simulink model "IEEE34BARRAS"  (R2018a)
settings: Solver=ode4  StartTime=0.0  StopTime=48*T  FixedStep=Ts  RelTol=1e-3  EnableMultiTasking=on
InitFcn:
  | close
  | clc
  | clear
  | n=2^8;
  | f=60;
  | T=1/f;
  | Ts=1/(f*n);
  | NT=18;
  | set_param('IEEE34BARRAS/EMISOR-RECEPTOR/TCP_IP_RX1/ESCRITURA', 'Value','[0,0,0,0,0,0,0,0,0,0,0,0,0,0,0,0,0,0,0,0,0,0,0,0,0,0,0,0,0,0,0,0,0,0,0,0,0,0,0,0,0]')
  | set_param('IEEE34BARRAS/EMISOR-RECEPTOR/TCP_IP_RX1/RETARDO', 'Value','0')
  | run script_client_1_inicio1.m
undefined symbols (not defined in the file or in its folder): D1, Delta, DiscIntNeverNeededParam, Ip1
libraries: powerlib x313, simulink x15, libreria_medidores1T x3, libreria_comunicaciones_cliente1T x2
(part 4 of 5)

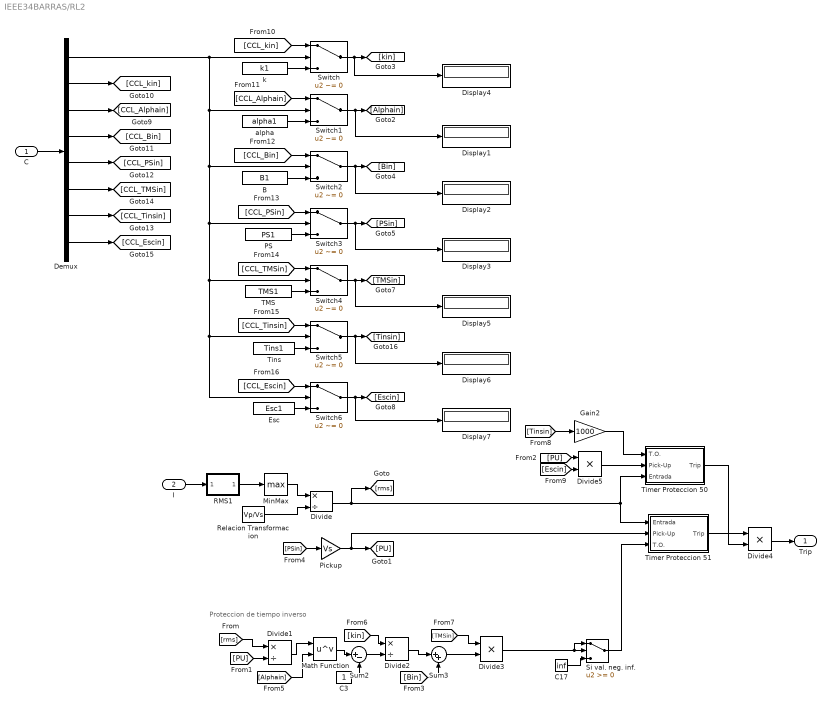
== system IEEE34BARRAS/RL2 ==
  note: Proteccion de tiempo inverso
  C : Inport
  I : Inport  Port=2
  B : Constant  Value=B1
  C17 : Constant  Value=inf
  C3 : Constant
  Demux : Demux  Outputs=8
  Display{1..7} (7 alike) : Display
  Divide : Product  Inputs=*/
  Divide1 : Product  Inputs=*/
  Divide2 : Product  Inputs=*/
  Divide3 : Product  Inputs=**
  Divide4 : Product  Inputs=**
  Divide5 : Product  Inputs=**
  Esc : Constant  Value=Esc1
  Gain2 : Gain  Gain=1000
  Math Function : Math  Operator=pow  SaturateOnIntegerOverflow=on
  MinMax : MinMax  Function=max
  PS : Constant  Value=PS1
  Pickup : Gain  Gain=Vs
  RMS1 : Subsystem
  Relacion Transformacion : Constant  Value=Vp/Vs
  Si val. neg. inf. : Switch
  Sum2 : Sum  Inputs=|+-
  Sum3 : Sum  Inputs=|++
  Switch{,1..6} (7 alike) : Switch  Criteria=u2 ~= 0
  TMS : Constant  Value=TMS1
  Timer Proteccion 50 : Subsystem
  Timer Proteccion 51 : Subsystem
  Tins : Constant  Value=Tins1
  alpha : Constant  Value=alpha1
  k : Constant  Value=k1
  Trip : Outport
  wires:
  Divide4/1 -> Trip/1
  [Escin] -> Divide5/2
  C17/1 -> Si val. neg. inf./3
  Math Function/1 -> Sum2/1
  [kin] -> Divide2/1
  Timer Proteccion 50/1(Trip) -> Divide4/2
  [PSin] -> Pickup/1
  Si val. neg. inf./1 -> Timer Proteccion 51/3(T.O.)
  [Tinsin] -> Gain2/1
  Timer Proteccion 51/1(Trip) -> Divide4/1
  [Alphain] -> Math Function/2
  [PU] -> Divide1/2
  [PU] -> Divide5/1
  Divide5/1 -> Timer Proteccion 50/2(Pick-Up)
  Divide2/1 -> Sum3/1
  Gain2/1 -> Timer Proteccion 50/1(T.O.)
  Divide3/1 -> Si val. neg. inf./1, Si val. neg. inf./2
  Sum3/1 -> Divide3/2
  [Bin] -> Sum3/2
  Relacion Transformacion/1 -> Divide/2
  Divide/1 -> Timer Proteccion 50/3(Entrada), Timer Proteccion 51/1(Entrada), [rms]
  Sum2/1 -> Divide2/2
  Divide1/1 -> Math Function/1
  [rms] -> Divide1/1
  Pickup/1 -> Timer Proteccion 51/2(Pick-Up), [PU]
  MinMax/1 -> Divide/1
  RMS1/1(Out1) -> MinMax/1
  [TMSin] -> Divide3/1
  C3/1 -> Sum2/2
  I/1 -> RMS1/1(In1)
  C/1 -> Demux/1
  Demux/1 -> Switch2/2, Switch4/2, Switch6/2, Switch5/2, Switch3/2, Switch1/2, Switch/2
  Demux/7 -> [CCL_Tinsin]
  Demux/5 -> [CCL_PSin]
  Demux/4 -> [CCL_Bin]
  Demux/2 -> [CCL_kin]
  Demux/3 -> [CCL_Alphain]
  Demux/6 -> [CCL_TMSin]
  Demux/8 -> [CCL_Escin]
  B/1 -> Switch2/3
  PS/1 -> Switch3/3
  TMS/1 -> Switch4/3
  Tins/1 -> Switch5/3
  Esc/1 -> Switch6/3
  Switch/1 -> Display4/1, [kin]
  Switch1/1 -> Display1/1, [Alphain]
  Switch3/1 -> Display3/1, [PSin]
  Switch4/1 -> Display5/1, [TMSin]
  Switch5/1 -> Display6/1, [Tinsin]
  Switch6/1 -> Display7/1, [Escin]
  alpha/1 -> Switch1/3
  [CCL_Alphain] -> Switch1/1
  [CCL_Bin] -> Switch2/1
  [CCL_PSin] -> Switch3/1
  [CCL_TMSin] -> Switch4/1
  [CCL_Tinsin] -> Switch5/1
  [CCL_Escin] -> Switch6/1
  k/1 -> Switch/3
  [CCL_kin] -> Switch/1
  Switch2/1 -> Display2/1, [Bin]

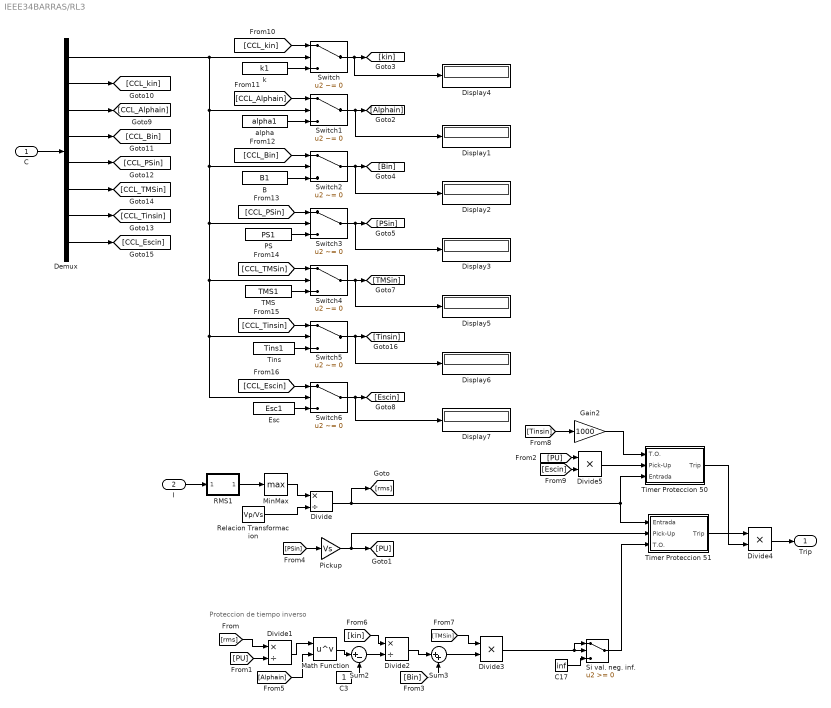
== system IEEE34BARRAS/RL3 ==
  note: Proteccion de tiempo inverso
  C : Inport
  I : Inport  Port=2
  B : Constant  Value=B1
  C17 : Constant  Value=inf
  C3 : Constant
  Demux : Demux  Outputs=8
  Display{1..7} (7 alike) : Display
  Divide : Product  Inputs=*/
  Divide1 : Product  Inputs=*/
  Divide2 : Product  Inputs=*/
  Divide3 : Product  Inputs=**
  Divide4 : Product  Inputs=**
  Divide5 : Product  Inputs=**
  Esc : Constant  Value=Esc1
  Gain2 : Gain  Gain=1000
  Math Function : Math  Operator=pow  SaturateOnIntegerOverflow=on
  MinMax : MinMax  Function=max
  PS : Constant  Value=PS1
  Pickup : Gain  Gain=Vs
  RMS1 : Subsystem
  Relacion Transformacion : Constant  Value=Vp/Vs
  Si val. neg. inf. : Switch
  Sum2 : Sum  Inputs=|+-
  Sum3 : Sum  Inputs=|++
  Switch{,1..6} (7 alike) : Switch  Criteria=u2 ~= 0
  TMS : Constant  Value=TMS1
  Timer Proteccion 50 : Subsystem
  Timer Proteccion 51 : Subsystem
  Tins : Constant  Value=Tins1
  alpha : Constant  Value=alpha1
  k : Constant  Value=k1
  Trip : Outport
  wires:
  Divide4/1 -> Trip/1
  [Escin] -> Divide5/2
  C17/1 -> Si val. neg. inf./3
  Math Function/1 -> Sum2/1
  [kin] -> Divide2/1
  Timer Proteccion 50/1(Trip) -> Divide4/2
  [PSin] -> Pickup/1
  Si val. neg. inf./1 -> Timer Proteccion 51/3(T.O.)
  [Tinsin] -> Gain2/1
  Timer Proteccion 51/1(Trip) -> Divide4/1
  [Alphain] -> Math Function/2
  [PU] -> Divide1/2
  [PU] -> Divide5/1
  Divide5/1 -> Timer Proteccion 50/2(Pick-Up)
  Divide2/1 -> Sum3/1
  Gain2/1 -> Timer Proteccion 50/1(T.O.)
  Divide3/1 -> Si val. neg. inf./1, Si val. neg. inf./2
  Sum3/1 -> Divide3/2
  [Bin] -> Sum3/2
  Relacion Transformacion/1 -> Divide/2
  Divide/1 -> Timer Proteccion 50/3(Entrada), Timer Proteccion 51/1(Entrada), [rms]
  Sum2/1 -> Divide2/2
  Divide1/1 -> Math Function/1
  [rms] -> Divide1/1
  Pickup/1 -> Timer Proteccion 51/2(Pick-Up), [PU]
  MinMax/1 -> Divide/1
  RMS1/1(Out1) -> MinMax/1
  [TMSin] -> Divide3/1
  C3/1 -> Sum2/2
  I/1 -> RMS1/1(In1)
  C/1 -> Demux/1
  Demux/1 -> Switch2/2, Switch4/2, Switch6/2, Switch5/2, Switch3/2, Switch1/2, Switch/2
  Demux/7 -> [CCL_Tinsin]
  Demux/5 -> [CCL_PSin]
  Demux/4 -> [CCL_Bin]
  Demux/2 -> [CCL_kin]
  Demux/3 -> [CCL_Alphain]
  Demux/6 -> [CCL_TMSin]
  Demux/8 -> [CCL_Escin]
  B/1 -> Switch2/3
  PS/1 -> Switch3/3
  TMS/1 -> Switch4/3
  Tins/1 -> Switch5/3
  Esc/1 -> Switch6/3
  Switch/1 -> Display4/1, [kin]
  Switch1/1 -> Display1/1, [Alphain]
  Switch3/1 -> Display3/1, [PSin]
  Switch4/1 -> Display5/1, [TMSin]
  Switch5/1 -> Display6/1, [Tinsin]
  Switch6/1 -> Display7/1, [Escin]
  alpha/1 -> Switch1/3
  [CCL_Alphain] -> Switch1/1
  [CCL_Bin] -> Switch2/1
  [CCL_PSin] -> Switch3/1
  [CCL_TMSin] -> Switch4/1
  [CCL_Tinsin] -> Switch5/1
  [CCL_Escin] -> Switch6/1
  k/1 -> Switch/3
  [CCL_kin] -> Switch/1
  Switch2/1 -> Display2/1, [Bin]

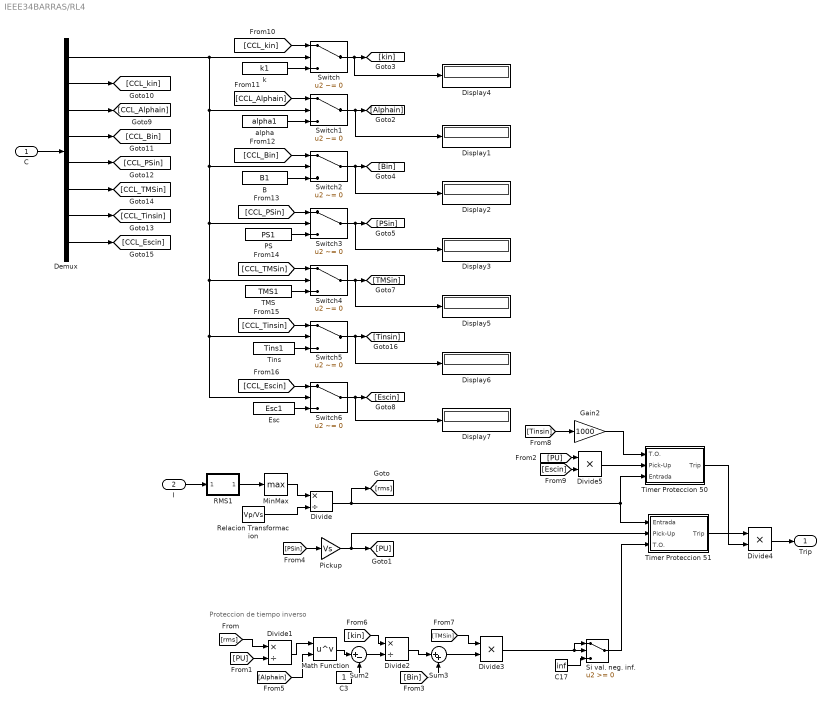
== system IEEE34BARRAS/RL4 ==
  note: Proteccion de tiempo inverso
  C : Inport
  I : Inport  Port=2
  B : Constant  Value=B1
  C17 : Constant  Value=inf
  C3 : Constant
  Demux : Demux  Outputs=8
  Display{1..7} (7 alike) : Display
  Divide : Product  Inputs=*/
  Divide1 : Product  Inputs=*/
  Divide2 : Product  Inputs=*/
  Divide3 : Product  Inputs=**
  Divide4 : Product  Inputs=**
  Divide5 : Product  Inputs=**
  Esc : Constant  Value=Esc1
  Gain2 : Gain  Gain=1000
  Math Function : Math  Operator=pow  SaturateOnIntegerOverflow=on
  MinMax : MinMax  Function=max
  PS : Constant  Value=PS1
  Pickup : Gain  Gain=Vs
  RMS1 : Subsystem
  Relacion Transformacion : Constant  Value=Vp/Vs
  Si val. neg. inf. : Switch
  Sum2 : Sum  Inputs=|+-
  Sum3 : Sum  Inputs=|++
  Switch{,1..6} (7 alike) : Switch  Criteria=u2 ~= 0
  TMS : Constant  Value=TMS1
  Timer Proteccion 50 : Subsystem
  Timer Proteccion 51 : Subsystem
  Tins : Constant  Value=Tins1
  alpha : Constant  Value=alpha1
  k : Constant  Value=k1
  Trip : Outport
  wires:
  Divide4/1 -> Trip/1
  [Escin] -> Divide5/2
  C17/1 -> Si val. neg. inf./3
  Math Function/1 -> Sum2/1
  [kin] -> Divide2/1
  Timer Proteccion 50/1(Trip) -> Divide4/2
  [PSin] -> Pickup/1
  Si val. neg. inf./1 -> Timer Proteccion 51/3(T.O.)
  [Tinsin] -> Gain2/1
  Timer Proteccion 51/1(Trip) -> Divide4/1
  [Alphain] -> Math Function/2
  [PU] -> Divide1/2
  [PU] -> Divide5/1
  Divide5/1 -> Timer Proteccion 50/2(Pick-Up)
  Divide2/1 -> Sum3/1
  Gain2/1 -> Timer Proteccion 50/1(T.O.)
  Divide3/1 -> Si val. neg. inf./1, Si val. neg. inf./2
  Sum3/1 -> Divide3/2
  [Bin] -> Sum3/2
  Relacion Transformacion/1 -> Divide/2
  Divide/1 -> Timer Proteccion 50/3(Entrada), Timer Proteccion 51/1(Entrada), [rms]
  Sum2/1 -> Divide2/2
  Divide1/1 -> Math Function/1
  [rms] -> Divide1/1
  Pickup/1 -> Timer Proteccion 51/2(Pick-Up), [PU]
  MinMax/1 -> Divide/1
  RMS1/1(Out1) -> MinMax/1
  [TMSin] -> Divide3/1
  C3/1 -> Sum2/2
  I/1 -> RMS1/1(In1)
  C/1 -> Demux/1
  Demux/1 -> Switch2/2, Switch4/2, Switch6/2, Switch5/2, Switch3/2, Switch1/2, Switch/2
  Demux/7 -> [CCL_Tinsin]
  Demux/5 -> [CCL_PSin]
  Demux/4 -> [CCL_Bin]
  Demux/2 -> [CCL_kin]
  Demux/3 -> [CCL_Alphain]
  Demux/6 -> [CCL_TMSin]
  Demux/8 -> [CCL_Escin]
  B/1 -> Switch2/3
  PS/1 -> Switch3/3
  TMS/1 -> Switch4/3
  Tins/1 -> Switch5/3
  Esc/1 -> Switch6/3
  Switch/1 -> Display4/1, [kin]
  Switch1/1 -> Display1/1, [Alphain]
  Switch3/1 -> Display3/1, [PSin]
  Switch4/1 -> Display5/1, [TMSin]
  Switch5/1 -> Display6/1, [Tinsin]
  Switch6/1 -> Display7/1, [Escin]
  alpha/1 -> Switch1/3
  [CCL_Alphain] -> Switch1/1
  [CCL_Bin] -> Switch2/1
  [CCL_PSin] -> Switch3/1
  [CCL_TMSin] -> Switch4/1
  [CCL_Tinsin] -> Switch5/1
  [CCL_Escin] -> Switch6/1
  k/1 -> Switch/3
  [CCL_kin] -> Switch/1
  Switch2/1 -> Display2/1, [Bin]

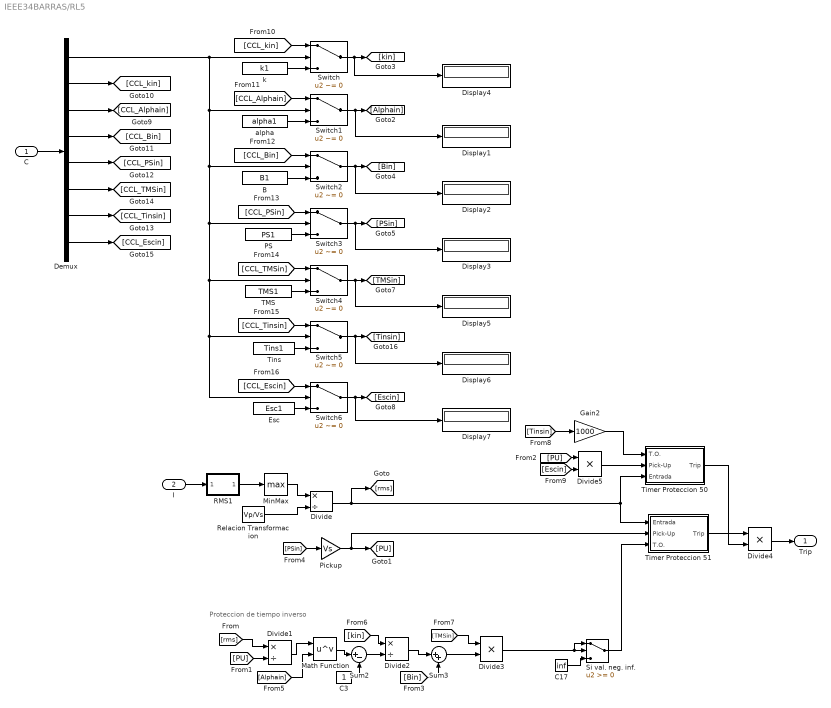
== system IEEE34BARRAS/RL5 ==
  note: Proteccion de tiempo inverso
  C : Inport
  I : Inport  Port=2
  B : Constant  Value=B1
  C17 : Constant  Value=inf
  C3 : Constant
  Demux : Demux  Outputs=8
  Display{1..7} (7 alike) : Display
  Divide : Product  Inputs=*/
  Divide1 : Product  Inputs=*/
  Divide2 : Product  Inputs=*/
  Divide3 : Product  Inputs=**
  Divide4 : Product  Inputs=**
  Divide5 : Product  Inputs=**
  Esc : Constant  Value=Esc1
  Gain2 : Gain  Gain=1000
  Math Function : Math  Operator=pow  SaturateOnIntegerOverflow=on
  MinMax : MinMax  Function=max
  PS : Constant  Value=PS1
  Pickup : Gain  Gain=Vs
  RMS1 : Subsystem
  Relacion Transformacion : Constant  Value=Vp/Vs
  Si val. neg. inf. : Switch
  Sum2 : Sum  Inputs=|+-
  Sum3 : Sum  Inputs=|++
  Switch{,1..6} (7 alike) : Switch  Criteria=u2 ~= 0
  TMS : Constant  Value=TMS1
  Timer Proteccion 50 : Subsystem
  Timer Proteccion 51 : Subsystem
  Tins : Constant  Value=Tins1
  alpha : Constant  Value=alpha1
  k : Constant  Value=k1
  Trip : Outport
  wires:
  Divide4/1 -> Trip/1
  [Escin] -> Divide5/2
  C17/1 -> Si val. neg. inf./3
  Math Function/1 -> Sum2/1
  [kin] -> Divide2/1
  Timer Proteccion 50/1(Trip) -> Divide4/2
  [PSin] -> Pickup/1
  Si val. neg. inf./1 -> Timer Proteccion 51/3(T.O.)
  [Tinsin] -> Gain2/1
  Timer Proteccion 51/1(Trip) -> Divide4/1
  [Alphain] -> Math Function/2
  [PU] -> Divide1/2
  [PU] -> Divide5/1
  Divide5/1 -> Timer Proteccion 50/2(Pick-Up)
  Divide2/1 -> Sum3/1
  Gain2/1 -> Timer Proteccion 50/1(T.O.)
  Divide3/1 -> Si val. neg. inf./1, Si val. neg. inf./2
  Sum3/1 -> Divide3/2
  [Bin] -> Sum3/2
  Relacion Transformacion/1 -> Divide/2
  Divide/1 -> Timer Proteccion 50/3(Entrada), Timer Proteccion 51/1(Entrada), [rms]
  Sum2/1 -> Divide2/2
  Divide1/1 -> Math Function/1
  [rms] -> Divide1/1
  Pickup/1 -> Timer Proteccion 51/2(Pick-Up), [PU]
  MinMax/1 -> Divide/1
  RMS1/1(Out1) -> MinMax/1
  [TMSin] -> Divide3/1
  C3/1 -> Sum2/2
  I/1 -> RMS1/1(In1)
  C/1 -> Demux/1
  Demux/1 -> Switch2/2, Switch4/2, Switch6/2, Switch5/2, Switch3/2, Switch1/2, Switch/2
  Demux/7 -> [CCL_Tinsin]
  Demux/5 -> [CCL_PSin]
  Demux/4 -> [CCL_Bin]
  Demux/2 -> [CCL_kin]
  Demux/3 -> [CCL_Alphain]
  Demux/6 -> [CCL_TMSin]
  Demux/8 -> [CCL_Escin]
  B/1 -> Switch2/3
  PS/1 -> Switch3/3
  TMS/1 -> Switch4/3
  Tins/1 -> Switch5/3
  Esc/1 -> Switch6/3
  Switch/1 -> Display4/1, [kin]
  Switch1/1 -> Display1/1, [Alphain]
  Switch3/1 -> Display3/1, [PSin]
  Switch4/1 -> Display5/1, [TMSin]
  Switch5/1 -> Display6/1, [Tinsin]
  Switch6/1 -> Display7/1, [Escin]
  alpha/1 -> Switch1/3
  [CCL_Alphain] -> Switch1/1
  [CCL_Bin] -> Switch2/1
  [CCL_PSin] -> Switch3/1
  [CCL_TMSin] -> Switch4/1
  [CCL_Tinsin] -> Switch5/1
  [CCL_Escin] -> Switch6/1
  k/1 -> Switch/3
  [CCL_kin] -> Switch/1
  Switch2/1 -> Display2/1, [Bin]

== system IEEE34BARRAS/Subsystem4 ==
  3p : powerlib/Elements/Three-Phase Fault  InitialStates=0  FaultA=on  FaultB=on  FaultC=on  GroundFault=on  SwitchTimes=[30*T]  External=off  SwitchStatus=NaN  FaultResistance=0.001  GroundResistance=1  SnubberResistance=1e6  SnubberCapacitance=inf  Measurements=None
  Conn1 : PMIOPort  Side=Left
  Conn2 : PMIOPort  Port=2  Side=Left
  Conn3 : PMIOPort  Port=3  Side=Left
  connections:
  3p/LConn3 -- Conn3/RConn1
  3p/LConn1 -- Conn1/RConn1
  3p/LConn2 -- Conn2/RConn1

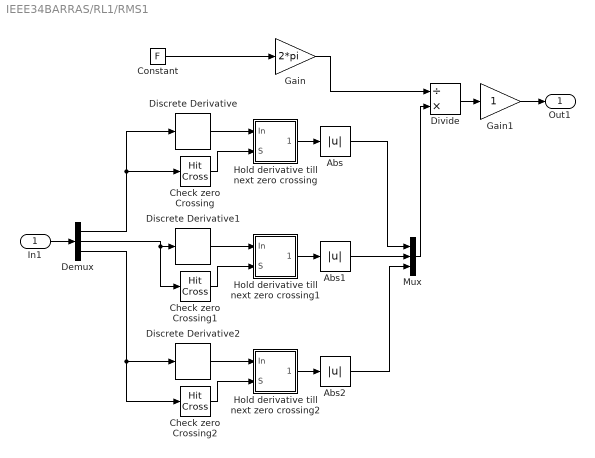
== system IEEE34BARRAS/RL1/RMS1 ==
  In1 : Inport
  Abs : Abs
  Abs1 : Abs
  Abs2 : Abs
  Check zero Crossing : HitCross
  Check zero Crossing1 : HitCross
  Check zero Crossing2 : HitCross
  Constant : Constant  Value=F
  Demux : Demux  Outputs=3
  Discrete Derivative : simulink/Discrete/Discrete Derivative  gainval=1.0  ICPrevScaledInput=0.0  OutMin=[]  OutMax=[]  OutDataType=fixdt(1, 16)  OutScaling=2^-10  DoSatur=off
  Discrete Derivative1 : simulink/Discrete/Discrete Derivative  gainval=1.0  ICPrevScaledInput=0.0  OutMin=[]  OutMax=[]  OutDataType=fixdt(1, 16)  OutScaling=2^-10  DoSatur=off
  Discrete Derivative2 : simulink/Discrete/Discrete Derivative  gainval=1.0  ICPrevScaledInput=0.0  OutMin=[]  OutMax=[]  OutDataType=fixdt(1, 16)  OutScaling=2^-10  DoSatur=off
  Divide : Product  Inputs=/*
  Gain : Gain  Gain=2*pi
  Gain1 : Gain
  Hold derivative till next zero crossing : Subsystem  AncestorBlock=|  DialogController=POWERSYS.PowerSysDialog  mask(Discrete Sample & Hold){ic=0, Ts=-1}
      | powerlib_extras/Discrete 
      | Control Blocks/Discrete
      | Sample & Hold
      mask prompts: ic "Initial condition:"; Ts "Sample time:"
      mask help: The output follows input 1 (In) as long as input 2 (S) is TRUE (1) . The output is held when input 2 becomes FALSE (0). The output initial value is specified by the parameter "Initial condition".
      mask init:
      | power_initmask();
      mask Help: This block is part of a subset of blocks in the Extras library that does not have documentation associated with it, other than the block mask description.
      mask Display: disp('S/H')
  Hold derivative till next zero crossing1 : Subsystem  AncestorBlock=|  DialogController=POWERSYS.PowerSysDialog  mask(Discrete Sample & Hold){ic=0, Ts=-1}
      | powerlib_extras/Discrete 
      | Control Blocks/Discrete
      | Sample & Hold
      mask prompts: ic "Initial condition:"; Ts "Sample time:"
      mask help: The output follows input 1 (In) as long as input 2 (S) is TRUE (1) . The output is held when input 2 becomes FALSE (0). The output initial value is specified by the parameter "Initial condition".
      mask init:
      | power_initmask();
      mask Help: This block is part of a subset of blocks in the Extras library that does not have documentation associated with it, other than the block mask description.
      mask Display: disp('S/H')
  Hold derivative till next zero crossing2 : Subsystem  AncestorBlock=|  DialogController=POWERSYS.PowerSysDialog  mask(Discrete Sample & Hold){ic=0, Ts=-1}
      | powerlib_extras/Discrete 
      | Control Blocks/Discrete
      | Sample & Hold
      mask prompts: ic "Initial condition:"; Ts "Sample time:"
      mask help: The output follows input 1 (In) as long as input 2 (S) is TRUE (1) . The output is held when input 2 becomes FALSE (0). The output initial value is specified by the parameter "Initial condition".
      mask init:
      | power_initmask();
      mask Help: This block is part of a subset of blocks in the Extras library that does not have documentation associated with it, other than the block mask description.
      mask Display: disp('S/H')
  Mux : Mux  Inputs=3
  Out1 : Outport
  wires:
  Discrete Derivative/1 -> Hold derivative till next zero crossing/1(In)
  Check zero Crossing/1 -> Hold derivative till next zero crossing/2(S)
  Hold derivative till next zero crossing/1("   ") -> Abs/1
  Constant/1 -> Gain/1
  Gain/1 -> Divide/1
  Abs/1 -> Mux/1
  Demux/1 -> Check zero Crossing/1, Discrete Derivative/1
  Divide/1 -> Gain1/1
  Gain1/1 -> Out1/1
  Hold derivative till next zero crossing1/1("   ") -> Abs1/1
  Check zero Crossing1/1 -> Hold derivative till next zero crossing1/2(S)
  Discrete Derivative1/1 -> Hold derivative till next zero crossing1/1(In)
  Discrete Derivative2/1 -> Hold derivative till next zero crossing2/1(In)
  Check zero Crossing2/1 -> Hold derivative till next zero crossing2/2(S)
  Hold derivative till next zero crossing2/1("   ") -> Abs2/1
  Demux/2 -> Check zero Crossing1/1, Discrete Derivative1/1
  Demux/3 -> Check zero Crossing2/1, Discrete Derivative2/1
  Abs1/1 -> Mux/2
  Mux/1 -> Divide/2
  Abs2/1 -> Mux/3
  In1/1 -> Demux/1

== system IEEE34BARRAS/RL1/Timer Proteccion 50 ==
  T.O. : Inport
  Pick-Up : Inport  Port=2
  Entrada : Inport  Port=3
  Arranq3 : Switch  Criteria=u2 ~= 0  Threshold=Ip1
  Arranq6 : Switch  Criteria=u2 ~= 0  Threshold=Ip1  ZeroCross=off
  C14 : Constant  Value=0
  C15 : Constant  Value=1000
  C16 : Constant
  Condicion arranque1 : RelationalOperator  Operator=>  OutDataTypeStr=boolean  RndMeth=Nearest
  Discrete-Time Integrator : DiscreteIntegrator  ExternalReset=falling  SampleTime=-1  ICPrevOutput=DiscIntNeverNeededParam  ICPrevScaledInput=DiscIntNeverNeededParam
  Logical Operator4 : Logic  Operator=NOT  AllPortsSameDT=off  OutDataTypeStr=boolean
  Tiempo Disparo1 : RelationalOperator  OutDataTypeStr=boolean  RndMeth=Nearest
  Trip : Outport
  wires:
  C16/1 -> Arranq6/1
  Arranq6/1 -> Logical Operator4/1, Arranq6/3
  Tiempo Disparo1/1 -> Arranq6/2
  C15/1 -> Arranq3/1
  C14/1 -> Arranq3/3
  Arranq3/1 -> Discrete-Time Integrator/1
  Condicion arranque1/1 -> Arranq3/2, Discrete-Time Integrator/2
  Pick-Up/1 -> Condicion arranque1/2
  Discrete-Time Integrator/1 -> Tiempo Disparo1/1
  Logical Operator4/1 -> Trip/1
  Entrada/1 -> Condicion arranque1/1
  T.O./1 -> Tiempo Disparo1/2

== system IEEE34BARRAS/RL1/Timer Proteccion 51 ==
  Entrada : Inport
  Pick-Up : Inport  Port=2
  T.O. : Inport  Port=3
  Arranq3 : Switch  Criteria=u2 ~= 0  Threshold=Ip1
  Arranq6 : Switch  Criteria=u2 ~= 0  Threshold=Ip1  ZeroCross=off
  C14 : Constant  Value=0
  C15 : Constant
  C16 : Constant
  Condicion arranque1 : RelationalOperator  Operator=>  OutDataTypeStr=boolean  RndMeth=Nearest
  Discrete-Time Integrator : DiscreteIntegrator  gainval=1  ExternalReset=falling  SampleTime=-1  ICPrevOutput=DiscIntNeverNeededParam  ICPrevScaledInput=DiscIntNeverNeededParam
  Logical Operator4 : Logic  Operator=NOT  AllPortsSameDT=off  OutDataTypeStr=boolean
  Tiempo Disparo1 : RelationalOperator  OutDataTypeStr=boolean  RndMeth=Nearest
  Trip : Outport
  wires:
  C16/1 -> Arranq6/1
  Arranq6/1 -> Logical Operator4/1, Arranq6/3
  Tiempo Disparo1/1 -> Arranq6/2
  T.O./1 -> Tiempo Disparo1/2
  C15/1 -> Arranq3/1
  C14/1 -> Arranq3/3
  Arranq3/1 -> Discrete-Time Integrator/1
  Condicion arranque1/1 -> Arranq3/2, Discrete-Time Integrator/2
  Pick-Up/1 -> Condicion arranque1/2
  Entrada/1 -> Condicion arranque1/1
  Discrete-Time Integrator/1 -> Tiempo Disparo1/1
  Logical Operator4/1 -> Trip/1

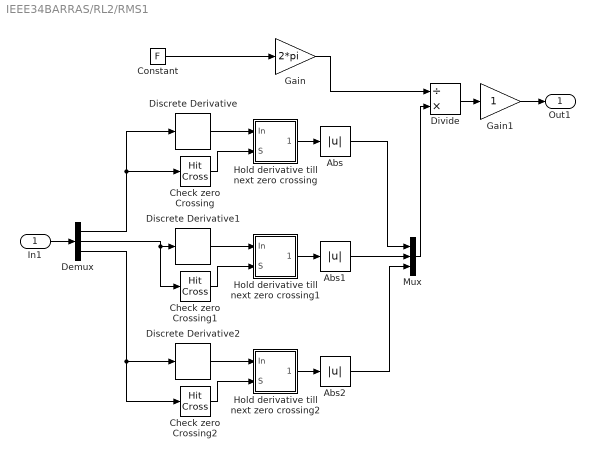
== system IEEE34BARRAS/RL2/RMS1 ==
  In1 : Inport
  Abs : Abs
  Abs1 : Abs
  Abs2 : Abs
  Check zero Crossing : HitCross
  Check zero Crossing1 : HitCross
  Check zero Crossing2 : HitCross
  Constant : Constant  Value=F
  Demux : Demux  Outputs=3
  Discrete Derivative : simulink/Discrete/Discrete Derivative  gainval=1.0  ICPrevScaledInput=0.0  OutMin=[]  OutMax=[]  OutDataType=fixdt(1, 16)  OutScaling=2^-10  DoSatur=off
  Discrete Derivative1 : simulink/Discrete/Discrete Derivative  gainval=1.0  ICPrevScaledInput=0.0  OutMin=[]  OutMax=[]  OutDataType=fixdt(1, 16)  OutScaling=2^-10  DoSatur=off
  Discrete Derivative2 : simulink/Discrete/Discrete Derivative  gainval=1.0  ICPrevScaledInput=0.0  OutMin=[]  OutMax=[]  OutDataType=fixdt(1, 16)  OutScaling=2^-10  DoSatur=off
  Divide : Product  Inputs=/*
  Gain : Gain  Gain=2*pi
  Gain1 : Gain
  Hold derivative till next zero crossing : Subsystem  AncestorBlock=|  DialogController=POWERSYS.PowerSysDialog  mask(Discrete Sample & Hold){ic=0, Ts=-1}
      | powerlib_extras/Discrete 
      | Control Blocks/Discrete
      | Sample & Hold
      mask prompts: ic "Initial condition:"; Ts "Sample time:"
      mask help: The output follows input 1 (In) as long as input 2 (S) is TRUE (1) . The output is held when input 2 becomes FALSE (0). The output initial value is specified by the parameter "Initial condition".
      mask init:
      | power_initmask();
      mask Help: This block is part of a subset of blocks in the Extras library that does not have documentation associated with it, other than the block mask description.
      mask Display: disp('S/H')
  Hold derivative till next zero crossing1 : Subsystem  AncestorBlock=|  DialogController=POWERSYS.PowerSysDialog  mask(Discrete Sample & Hold){ic=0, Ts=-1}
      | powerlib_extras/Discrete 
      | Control Blocks/Discrete
      | Sample & Hold
      mask prompts: ic "Initial condition:"; Ts "Sample time:"
      mask help: The output follows input 1 (In) as long as input 2 (S) is TRUE (1) . The output is held when input 2 becomes FALSE (0). The output initial value is specified by the parameter "Initial condition".
      mask init:
      | power_initmask();
      mask Help: This block is part of a subset of blocks in the Extras library that does not have documentation associated with it, other than the block mask description.
      mask Display: disp('S/H')
  Hold derivative till next zero crossing2 : Subsystem  AncestorBlock=|  DialogController=POWERSYS.PowerSysDialog  mask(Discrete Sample & Hold){ic=0, Ts=-1}
      | powerlib_extras/Discrete 
      | Control Blocks/Discrete
      | Sample & Hold
      mask prompts: ic "Initial condition:"; Ts "Sample time:"
      mask help: The output follows input 1 (In) as long as input 2 (S) is TRUE (1) . The output is held when input 2 becomes FALSE (0). The output initial value is specified by the parameter "Initial condition".
      mask init:
      | power_initmask();
      mask Help: This block is part of a subset of blocks in the Extras library that does not have documentation associated with it, other than the block mask description.
      mask Display: disp('S/H')
  Mux : Mux  Inputs=3
  Out1 : Outport
  wires:
  Discrete Derivative/1 -> Hold derivative till next zero crossing/1(In)
  Check zero Crossing/1 -> Hold derivative till next zero crossing/2(S)
  Hold derivative till next zero crossing/1("   ") -> Abs/1
  Constant/1 -> Gain/1
  Gain/1 -> Divide/1
  Abs/1 -> Mux/1
  Demux/1 -> Check zero Crossing/1, Discrete Derivative/1
  Divide/1 -> Gain1/1
  Gain1/1 -> Out1/1
  Hold derivative till next zero crossing1/1("   ") -> Abs1/1
  Check zero Crossing1/1 -> Hold derivative till next zero crossing1/2(S)
  Discrete Derivative1/1 -> Hold derivative till next zero crossing1/1(In)
  Discrete Derivative2/1 -> Hold derivative till next zero crossing2/1(In)
  Check zero Crossing2/1 -> Hold derivative till next zero crossing2/2(S)
  Hold derivative till next zero crossing2/1("   ") -> Abs2/1
  Demux/2 -> Check zero Crossing1/1, Discrete Derivative1/1
  Demux/3 -> Check zero Crossing2/1, Discrete Derivative2/1
  Abs1/1 -> Mux/2
  Mux/1 -> Divide/2
  Abs2/1 -> Mux/3
  In1/1 -> Demux/1

== system IEEE34BARRAS/RL2/Timer Proteccion 50 ==
  T.O. : Inport
  Pick-Up : Inport  Port=2
  Entrada : Inport  Port=3
  Arranq3 : Switch  Criteria=u2 ~= 0  Threshold=Ip1
  Arranq6 : Switch  Criteria=u2 ~= 0  Threshold=Ip1  ZeroCross=off
  C14 : Constant  Value=0
  C15 : Constant  Value=1000
  C16 : Constant
  Condicion arranque1 : RelationalOperator  Operator=>  OutDataTypeStr=boolean  RndMeth=Nearest
  Discrete-Time Integrator : DiscreteIntegrator  ExternalReset=falling  SampleTime=-1  ICPrevOutput=DiscIntNeverNeededParam  ICPrevScaledInput=DiscIntNeverNeededParam
  Logical Operator4 : Logic  Operator=NOT  AllPortsSameDT=off  OutDataTypeStr=boolean
  Tiempo Disparo1 : RelationalOperator  OutDataTypeStr=boolean  RndMeth=Nearest
  Trip : Outport
  wires:
  C16/1 -> Arranq6/1
  Arranq6/1 -> Logical Operator4/1, Arranq6/3
  Tiempo Disparo1/1 -> Arranq6/2
  C15/1 -> Arranq3/1
  C14/1 -> Arranq3/3
  Arranq3/1 -> Discrete-Time Integrator/1
  Condicion arranque1/1 -> Arranq3/2, Discrete-Time Integrator/2
  Pick-Up/1 -> Condicion arranque1/2
  Discrete-Time Integrator/1 -> Tiempo Disparo1/1
  Logical Operator4/1 -> Trip/1
  Entrada/1 -> Condicion arranque1/1
  T.O./1 -> Tiempo Disparo1/2

== system IEEE34BARRAS/RL2/Timer Proteccion 51 ==
  Entrada : Inport
  Pick-Up : Inport  Port=2
  T.O. : Inport  Port=3
  Arranq3 : Switch  Criteria=u2 ~= 0  Threshold=Ip1
  Arranq6 : Switch  Criteria=u2 ~= 0  Threshold=Ip1  ZeroCross=off
  C14 : Constant  Value=0
  C15 : Constant
  C16 : Constant
  Condicion arranque1 : RelationalOperator  Operator=>  OutDataTypeStr=boolean  RndMeth=Nearest
  Discrete-Time Integrator : DiscreteIntegrator  gainval=1  ExternalReset=falling  SampleTime=-1  ICPrevOutput=DiscIntNeverNeededParam  ICPrevScaledInput=DiscIntNeverNeededParam
  Logical Operator4 : Logic  Operator=NOT  AllPortsSameDT=off  OutDataTypeStr=boolean
  Tiempo Disparo1 : RelationalOperator  OutDataTypeStr=boolean  RndMeth=Nearest
  Trip : Outport
  wires:
  C16/1 -> Arranq6/1
  Arranq6/1 -> Logical Operator4/1, Arranq6/3
  Tiempo Disparo1/1 -> Arranq6/2
  T.O./1 -> Tiempo Disparo1/2
  C15/1 -> Arranq3/1
  C14/1 -> Arranq3/3
  Arranq3/1 -> Discrete-Time Integrator/1
  Condicion arranque1/1 -> Arranq3/2, Discrete-Time Integrator/2
  Pick-Up/1 -> Condicion arranque1/2
  Entrada/1 -> Condicion arranque1/1
  Discrete-Time Integrator/1 -> Tiempo Disparo1/1
  Logical Operator4/1 -> Trip/1

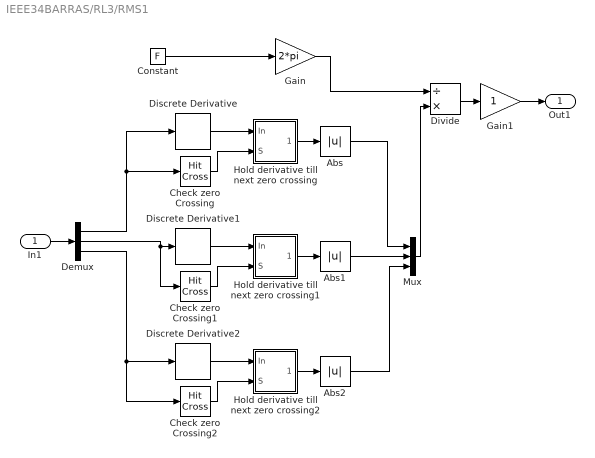
== system IEEE34BARRAS/RL3/RMS1 ==
  In1 : Inport
  Abs : Abs
  Abs1 : Abs
  Abs2 : Abs
  Check zero Crossing : HitCross
  Check zero Crossing1 : HitCross
  Check zero Crossing2 : HitCross
  Constant : Constant  Value=F
  Demux : Demux  Outputs=3
  Discrete Derivative : simulink/Discrete/Discrete Derivative  gainval=1.0  ICPrevScaledInput=0.0  OutMin=[]  OutMax=[]  OutDataType=fixdt(1, 16)  OutScaling=2^-10  DoSatur=off
  Discrete Derivative1 : simulink/Discrete/Discrete Derivative  gainval=1.0  ICPrevScaledInput=0.0  OutMin=[]  OutMax=[]  OutDataType=fixdt(1, 16)  OutScaling=2^-10  DoSatur=off
  Discrete Derivative2 : simulink/Discrete/Discrete Derivative  gainval=1.0  ICPrevScaledInput=0.0  OutMin=[]  OutMax=[]  OutDataType=fixdt(1, 16)  OutScaling=2^-10  DoSatur=off
  Divide : Product  Inputs=/*
  Gain : Gain  Gain=2*pi
  Gain1 : Gain
  Hold derivative till next zero crossing : Subsystem  AncestorBlock=|  DialogController=POWERSYS.PowerSysDialog  mask(Discrete Sample & Hold){ic=0, Ts=-1}
      | powerlib_extras/Discrete 
      | Control Blocks/Discrete
      | Sample & Hold
      mask prompts: ic "Initial condition:"; Ts "Sample time:"
      mask help: The output follows input 1 (In) as long as input 2 (S) is TRUE (1) . The output is held when input 2 becomes FALSE (0). The output initial value is specified by the parameter "Initial condition".
      mask init:
      | power_initmask();
      mask Help: This block is part of a subset of blocks in the Extras library that does not have documentation associated with it, other than the block mask description.
      mask Display: disp('S/H')
  Hold derivative till next zero crossing1 : Subsystem  AncestorBlock=|  DialogController=POWERSYS.PowerSysDialog  mask(Discrete Sample & Hold){ic=0, Ts=-1}
      | powerlib_extras/Discrete 
      | Control Blocks/Discrete
      | Sample & Hold
      mask prompts: ic "Initial condition:"; Ts "Sample time:"
      mask help: The output follows input 1 (In) as long as input 2 (S) is TRUE (1) . The output is held when input 2 becomes FALSE (0). The output initial value is specified by the parameter "Initial condition".
      mask init:
      | power_initmask();
      mask Help: This block is part of a subset of blocks in the Extras library that does not have documentation associated with it, other than the block mask description.
      mask Display: disp('S/H')
  Hold derivative till next zero crossing2 : Subsystem  AncestorBlock=|  DialogController=POWERSYS.PowerSysDialog  mask(Discrete Sample & Hold){ic=0, Ts=-1}
      | powerlib_extras/Discrete 
      | Control Blocks/Discrete
      | Sample & Hold
      mask prompts: ic "Initial condition:"; Ts "Sample time:"
      mask help: The output follows input 1 (In) as long as input 2 (S) is TRUE (1) . The output is held when input 2 becomes FALSE (0). The output initial value is specified by the parameter "Initial condition".
      mask init:
      | power_initmask();
      mask Help: This block is part of a subset of blocks in the Extras library that does not have documentation associated with it, other than the block mask description.
      mask Display: disp('S/H')
  Mux : Mux  Inputs=3
  Out1 : Outport
  wires:
  Discrete Derivative/1 -> Hold derivative till next zero crossing/1(In)
  Check zero Crossing/1 -> Hold derivative till next zero crossing/2(S)
  Hold derivative till next zero crossing/1("   ") -> Abs/1
  Constant/1 -> Gain/1
  Gain/1 -> Divide/1
  Abs/1 -> Mux/1
  Demux/1 -> Check zero Crossing/1, Discrete Derivative/1
  Divide/1 -> Gain1/1
  Gain1/1 -> Out1/1
  Hold derivative till next zero crossing1/1("   ") -> Abs1/1
  Check zero Crossing1/1 -> Hold derivative till next zero crossing1/2(S)
  Discrete Derivative1/1 -> Hold derivative till next zero crossing1/1(In)
  Discrete Derivative2/1 -> Hold derivative till next zero crossing2/1(In)
  Check zero Crossing2/1 -> Hold derivative till next zero crossing2/2(S)
  Hold derivative till next zero crossing2/1("   ") -> Abs2/1
  Demux/2 -> Check zero Crossing1/1, Discrete Derivative1/1
  Demux/3 -> Check zero Crossing2/1, Discrete Derivative2/1
  Abs1/1 -> Mux/2
  Mux/1 -> Divide/2
  Abs2/1 -> Mux/3
  In1/1 -> Demux/1

== system IEEE34BARRAS/RL3/Timer Proteccion 50 ==
  T.O. : Inport
  Pick-Up : Inport  Port=2
  Entrada : Inport  Port=3
  Arranq3 : Switch  Criteria=u2 ~= 0  Threshold=Ip1
  Arranq6 : Switch  Criteria=u2 ~= 0  Threshold=Ip1  ZeroCross=off
  C14 : Constant  Value=0
  C15 : Constant  Value=1000
  C16 : Constant
  Condicion arranque1 : RelationalOperator  Operator=>  OutDataTypeStr=boolean  RndMeth=Nearest
  Discrete-Time Integrator : DiscreteIntegrator  ExternalReset=falling  SampleTime=-1  ICPrevOutput=DiscIntNeverNeededParam  ICPrevScaledInput=DiscIntNeverNeededParam
  Logical Operator4 : Logic  Operator=NOT  AllPortsSameDT=off  OutDataTypeStr=boolean
  Tiempo Disparo1 : RelationalOperator  OutDataTypeStr=boolean  RndMeth=Nearest
  Trip : Outport
  wires:
  C16/1 -> Arranq6/1
  Arranq6/1 -> Logical Operator4/1, Arranq6/3
  Tiempo Disparo1/1 -> Arranq6/2
  C15/1 -> Arranq3/1
  C14/1 -> Arranq3/3
  Arranq3/1 -> Discrete-Time Integrator/1
  Condicion arranque1/1 -> Arranq3/2, Discrete-Time Integrator/2
  Pick-Up/1 -> Condicion arranque1/2
  Discrete-Time Integrator/1 -> Tiempo Disparo1/1
  Logical Operator4/1 -> Trip/1
  Entrada/1 -> Condicion arranque1/1
  T.O./1 -> Tiempo Disparo1/2

== system IEEE34BARRAS/RL3/Timer Proteccion 51 ==
  Entrada : Inport
  Pick-Up : Inport  Port=2
  T.O. : Inport  Port=3
  Arranq3 : Switch  Criteria=u2 ~= 0  Threshold=Ip1
  Arranq6 : Switch  Criteria=u2 ~= 0  Threshold=Ip1  ZeroCross=off
  C14 : Constant  Value=0
  C15 : Constant
  C16 : Constant
  Condicion arranque1 : RelationalOperator  Operator=>  OutDataTypeStr=boolean  RndMeth=Nearest
  Discrete-Time Integrator : DiscreteIntegrator  gainval=1  ExternalReset=falling  SampleTime=-1  ICPrevOutput=DiscIntNeverNeededParam  ICPrevScaledInput=DiscIntNeverNeededParam
  Logical Operator4 : Logic  Operator=NOT  AllPortsSameDT=off  OutDataTypeStr=boolean
  Tiempo Disparo1 : RelationalOperator  OutDataTypeStr=boolean  RndMeth=Nearest
  Trip : Outport
  wires:
  C16/1 -> Arranq6/1
  Arranq6/1 -> Logical Operator4/1, Arranq6/3
  Tiempo Disparo1/1 -> Arranq6/2
  T.O./1 -> Tiempo Disparo1/2
  C15/1 -> Arranq3/1
  C14/1 -> Arranq3/3
  Arranq3/1 -> Discrete-Time Integrator/1
  Condicion arranque1/1 -> Arranq3/2, Discrete-Time Integrator/2
  Pick-Up/1 -> Condicion arranque1/2
  Entrada/1 -> Condicion arranque1/1
  Discrete-Time Integrator/1 -> Tiempo Disparo1/1
  Logical Operator4/1 -> Trip/1

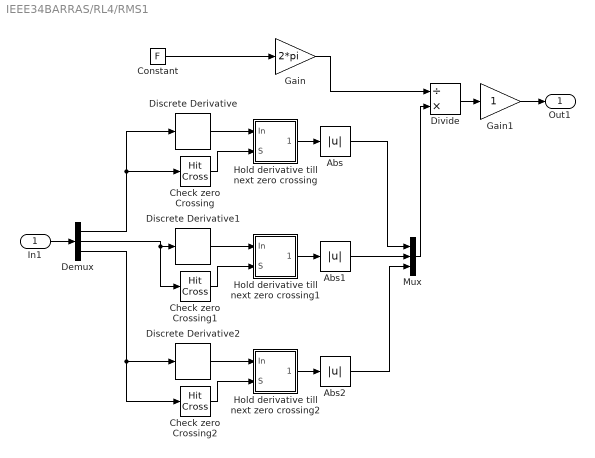
== system IEEE34BARRAS/RL4/RMS1 ==
  In1 : Inport
  Abs : Abs
  Abs1 : Abs
  Abs2 : Abs
  Check zero Crossing : HitCross
  Check zero Crossing1 : HitCross
  Check zero Crossing2 : HitCross
  Constant : Constant  Value=F
  Demux : Demux  Outputs=3
  Discrete Derivative : simulink/Discrete/Discrete Derivative  gainval=1.0  ICPrevScaledInput=0.0  OutMin=[]  OutMax=[]  OutDataType=fixdt(1, 16)  OutScaling=2^-10  DoSatur=off
  Discrete Derivative1 : simulink/Discrete/Discrete Derivative  gainval=1.0  ICPrevScaledInput=0.0  OutMin=[]  OutMax=[]  OutDataType=fixdt(1, 16)  OutScaling=2^-10  DoSatur=off
  Discrete Derivative2 : simulink/Discrete/Discrete Derivative  gainval=1.0  ICPrevScaledInput=0.0  OutMin=[]  OutMax=[]  OutDataType=fixdt(1, 16)  OutScaling=2^-10  DoSatur=off
  Divide : Product  Inputs=/*
  Gain : Gain  Gain=2*pi
  Gain1 : Gain
  Hold derivative till next zero crossing : Subsystem  AncestorBlock=|  DialogController=POWERSYS.PowerSysDialog  mask(Discrete Sample & Hold){ic=0, Ts=-1}
      | powerlib_extras/Discrete 
      | Control Blocks/Discrete
      | Sample & Hold
      mask prompts: ic "Initial condition:"; Ts "Sample time:"
      mask help: The output follows input 1 (In) as long as input 2 (S) is TRUE (1) . The output is held when input 2 becomes FALSE (0). The output initial value is specified by the parameter "Initial condition".
      mask init:
      | power_initmask();
      mask Help: This block is part of a subset of blocks in the Extras library that does not have documentation associated with it, other than the block mask description.
      mask Display: disp('S/H')
  Hold derivative till next zero crossing1 : Subsystem  AncestorBlock=|  DialogController=POWERSYS.PowerSysDialog  mask(Discrete Sample & Hold){ic=0, Ts=-1}
      | powerlib_extras/Discrete 
      | Control Blocks/Discrete
      | Sample & Hold
      mask prompts: ic "Initial condition:"; Ts "Sample time:"
      mask help: The output follows input 1 (In) as long as input 2 (S) is TRUE (1) . The output is held when input 2 becomes FALSE (0). The output initial value is specified by the parameter "Initial condition".
      mask init:
      | power_initmask();
      mask Help: This block is part of a subset of blocks in the Extras library that does not have documentation associated with it, other than the block mask description.
      mask Display: disp('S/H')
  Hold derivative till next zero crossing2 : Subsystem  AncestorBlock=|  DialogController=POWERSYS.PowerSysDialog  mask(Discrete Sample & Hold){ic=0, Ts=-1}
      | powerlib_extras/Discrete 
      | Control Blocks/Discrete
      | Sample & Hold
      mask prompts: ic "Initial condition:"; Ts "Sample time:"
      mask help: The output follows input 1 (In) as long as input 2 (S) is TRUE (1) . The output is held when input 2 becomes FALSE (0). The output initial value is specified by the parameter "Initial condition".
      mask init:
      | power_initmask();
      mask Help: This block is part of a subset of blocks in the Extras library that does not have documentation associated with it, other than the block mask description.
      mask Display: disp('S/H')
  Mux : Mux  Inputs=3
  Out1 : Outport
  wires:
  Discrete Derivative/1 -> Hold derivative till next zero crossing/1(In)
  Check zero Crossing/1 -> Hold derivative till next zero crossing/2(S)
  Hold derivative till next zero crossing/1("   ") -> Abs/1
  Constant/1 -> Gain/1
  Gain/1 -> Divide/1
  Abs/1 -> Mux/1
  Demux/1 -> Check zero Crossing/1, Discrete Derivative/1
  Divide/1 -> Gain1/1
  Gain1/1 -> Out1/1
  Hold derivative till next zero crossing1/1("   ") -> Abs1/1
  Check zero Crossing1/1 -> Hold derivative till next zero crossing1/2(S)
  Discrete Derivative1/1 -> Hold derivative till next zero crossing1/1(In)
  Discrete Derivative2/1 -> Hold derivative till next zero crossing2/1(In)
  Check zero Crossing2/1 -> Hold derivative till next zero crossing2/2(S)
  Hold derivative till next zero crossing2/1("   ") -> Abs2/1
  Demux/2 -> Check zero Crossing1/1, Discrete Derivative1/1
  Demux/3 -> Check zero Crossing2/1, Discrete Derivative2/1
  Abs1/1 -> Mux/2
  Mux/1 -> Divide/2
  Abs2/1 -> Mux/3
  In1/1 -> Demux/1

== system IEEE34BARRAS/RL4/Timer Proteccion 50 ==
  T.O. : Inport
  Pick-Up : Inport  Port=2
  Entrada : Inport  Port=3
  Arranq3 : Switch  Criteria=u2 ~= 0  Threshold=Ip1
  Arranq6 : Switch  Criteria=u2 ~= 0  Threshold=Ip1  ZeroCross=off
  C14 : Constant  Value=0
  C15 : Constant  Value=1000
  C16 : Constant
  Condicion arranque1 : RelationalOperator  Operator=>  OutDataTypeStr=boolean  RndMeth=Nearest
  Discrete-Time Integrator : DiscreteIntegrator  ExternalReset=falling  SampleTime=-1  ICPrevOutput=DiscIntNeverNeededParam  ICPrevScaledInput=DiscIntNeverNeededParam
  Logical Operator4 : Logic  Operator=NOT  AllPortsSameDT=off  OutDataTypeStr=boolean
  Tiempo Disparo1 : RelationalOperator  OutDataTypeStr=boolean  RndMeth=Nearest
  Trip : Outport
  wires:
  C16/1 -> Arranq6/1
  Arranq6/1 -> Logical Operator4/1, Arranq6/3
  Tiempo Disparo1/1 -> Arranq6/2
  C15/1 -> Arranq3/1
  C14/1 -> Arranq3/3
  Arranq3/1 -> Discrete-Time Integrator/1
  Condicion arranque1/1 -> Arranq3/2, Discrete-Time Integrator/2
  Pick-Up/1 -> Condicion arranque1/2
  Discrete-Time Integrator/1 -> Tiempo Disparo1/1
  Logical Operator4/1 -> Trip/1
  Entrada/1 -> Condicion arranque1/1
  T.O./1 -> Tiempo Disparo1/2

== system IEEE34BARRAS/RL4/Timer Proteccion 51 ==
  Entrada : Inport
  Pick-Up : Inport  Port=2
  T.O. : Inport  Port=3
  Arranq3 : Switch  Criteria=u2 ~= 0  Threshold=Ip1
  Arranq6 : Switch  Criteria=u2 ~= 0  Threshold=Ip1  ZeroCross=off
  C14 : Constant  Value=0
  C15 : Constant
  C16 : Constant
  Condicion arranque1 : RelationalOperator  Operator=>  OutDataTypeStr=boolean  RndMeth=Nearest
  Discrete-Time Integrator : DiscreteIntegrator  gainval=1  ExternalReset=falling  SampleTime=-1  ICPrevOutput=DiscIntNeverNeededParam  ICPrevScaledInput=DiscIntNeverNeededParam
  Logical Operator4 : Logic  Operator=NOT  AllPortsSameDT=off  OutDataTypeStr=boolean
  Tiempo Disparo1 : RelationalOperator  OutDataTypeStr=boolean  RndMeth=Nearest
  Trip : Outport
  wires:
  C16/1 -> Arranq6/1
  Arranq6/1 -> Logical Operator4/1, Arranq6/3
  Tiempo Disparo1/1 -> Arranq6/2
  T.O./1 -> Tiempo Disparo1/2
  C15/1 -> Arranq3/1
  C14/1 -> Arranq3/3
  Arranq3/1 -> Discrete-Time Integrator/1
  Condicion arranque1/1 -> Arranq3/2, Discrete-Time Integrator/2
  Pick-Up/1 -> Condicion arranque1/2
  Entrada/1 -> Condicion arranque1/1
  Discrete-Time Integrator/1 -> Tiempo Disparo1/1
  Logical Operator4/1 -> Trip/1

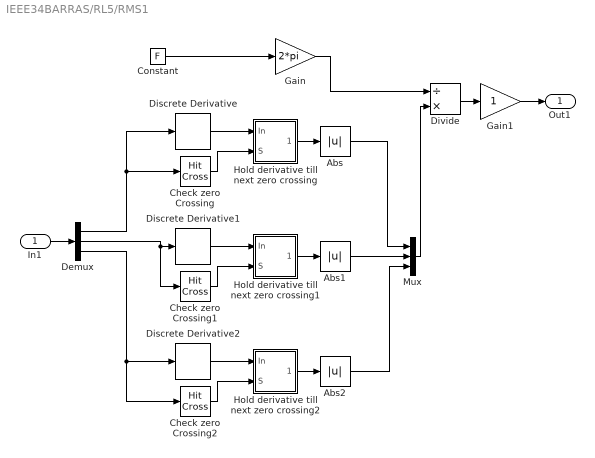
== system IEEE34BARRAS/RL5/RMS1 ==
  In1 : Inport
  Abs : Abs
  Abs1 : Abs
  Abs2 : Abs
  Check zero Crossing : HitCross
  Check zero Crossing1 : HitCross
  Check zero Crossing2 : HitCross
  Constant : Constant  Value=F
  Demux : Demux  Outputs=3
  Discrete Derivative : simulink/Discrete/Discrete Derivative  gainval=1.0  ICPrevScaledInput=0.0  OutMin=[]  OutMax=[]  OutDataType=fixdt(1, 16)  OutScaling=2^-10  DoSatur=off
  Discrete Derivative1 : simulink/Discrete/Discrete Derivative  gainval=1.0  ICPrevScaledInput=0.0  OutMin=[]  OutMax=[]  OutDataType=fixdt(1, 16)  OutScaling=2^-10  DoSatur=off
  Discrete Derivative2 : simulink/Discrete/Discrete Derivative  gainval=1.0  ICPrevScaledInput=0.0  OutMin=[]  OutMax=[]  OutDataType=fixdt(1, 16)  OutScaling=2^-10  DoSatur=off
  Divide : Product  Inputs=/*
  Gain : Gain  Gain=2*pi
  Gain1 : Gain
  Hold derivative till next zero crossing : Subsystem  AncestorBlock=|  DialogController=POWERSYS.PowerSysDialog  mask(Discrete Sample & Hold){ic=0, Ts=-1}
      | powerlib_extras/Discrete 
      | Control Blocks/Discrete
      | Sample & Hold
      mask prompts: ic "Initial condition:"; Ts "Sample time:"
      mask help: The output follows input 1 (In) as long as input 2 (S) is TRUE (1) . The output is held when input 2 becomes FALSE (0). The output initial value is specified by the parameter "Initial condition".
      mask init:
      | power_initmask();
      mask Help: This block is part of a subset of blocks in the Extras library that does not have documentation associated with it, other than the block mask description.
      mask Display: disp('S/H')
  Hold derivative till next zero crossing1 : Subsystem  AncestorBlock=|  DialogController=POWERSYS.PowerSysDialog  mask(Discrete Sample & Hold){ic=0, Ts=-1}
      | powerlib_extras/Discrete 
      | Control Blocks/Discrete
      | Sample & Hold
      mask prompts: ic "Initial condition:"; Ts "Sample time:"
      mask help: The output follows input 1 (In) as long as input 2 (S) is TRUE (1) . The output is held when input 2 becomes FALSE (0). The output initial value is specified by the parameter "Initial condition".
      mask init:
      | power_initmask();
      mask Help: This block is part of a subset of blocks in the Extras library that does not have documentation associated with it, other than the block mask description.
      mask Display: disp('S/H')
  Hold derivative till next zero crossing2 : Subsystem  AncestorBlock=|  DialogController=POWERSYS.PowerSysDialog  mask(Discrete Sample & Hold){ic=0, Ts=-1}
      | powerlib_extras/Discrete 
      | Control Blocks/Discrete
      | Sample & Hold
      mask prompts: ic "Initial condition:"; Ts "Sample time:"
      mask help: The output follows input 1 (In) as long as input 2 (S) is TRUE (1) . The output is held when input 2 becomes FALSE (0). The output initial value is specified by the parameter "Initial condition".
      mask init:
      | power_initmask();
      mask Help: This block is part of a subset of blocks in the Extras library that does not have documentation associated with it, other than the block mask description.
      mask Display: disp('S/H')
  Mux : Mux  Inputs=3
  Out1 : Outport
  wires:
  Discrete Derivative/1 -> Hold derivative till next zero crossing/1(In)
  Check zero Crossing/1 -> Hold derivative till next zero crossing/2(S)
  Hold derivative till next zero crossing/1("   ") -> Abs/1
  Constant/1 -> Gain/1
  Gain/1 -> Divide/1
  Abs/1 -> Mux/1
  Demux/1 -> Check zero Crossing/1, Discrete Derivative/1
  Divide/1 -> Gain1/1
  Gain1/1 -> Out1/1
  Hold derivative till next zero crossing1/1("   ") -> Abs1/1
  Check zero Crossing1/1 -> Hold derivative till next zero crossing1/2(S)
  Discrete Derivative1/1 -> Hold derivative till next zero crossing1/1(In)
  Discrete Derivative2/1 -> Hold derivative till next zero crossing2/1(In)
  Check zero Crossing2/1 -> Hold derivative till next zero crossing2/2(S)
  Hold derivative till next zero crossing2/1("   ") -> Abs2/1
  Demux/2 -> Check zero Crossing1/1, Discrete Derivative1/1
  Demux/3 -> Check zero Crossing2/1, Discrete Derivative2/1
  Abs1/1 -> Mux/2
  Mux/1 -> Divide/2
  Abs2/1 -> Mux/3
  In1/1 -> Demux/1

== system IEEE34BARRAS/RL5/Timer Proteccion 50 ==
  T.O. : Inport
  Pick-Up : Inport  Port=2
  Entrada : Inport  Port=3
  Arranq3 : Switch  Criteria=u2 ~= 0  Threshold=Ip1
  Arranq6 : Switch  Criteria=u2 ~= 0  Threshold=Ip1  ZeroCross=off
  C14 : Constant  Value=0
  C15 : Constant  Value=1000
  C16 : Constant
  Condicion arranque1 : RelationalOperator  Operator=>  OutDataTypeStr=boolean  RndMeth=Nearest
  Discrete-Time Integrator : DiscreteIntegrator  ExternalReset=falling  SampleTime=-1  ICPrevOutput=DiscIntNeverNeededParam  ICPrevScaledInput=DiscIntNeverNeededParam
  Logical Operator4 : Logic  Operator=NOT  AllPortsSameDT=off  OutDataTypeStr=boolean
  Tiempo Disparo1 : RelationalOperator  OutDataTypeStr=boolean  RndMeth=Nearest
  Trip : Outport
  wires:
  C16/1 -> Arranq6/1
  Arranq6/1 -> Logical Operator4/1, Arranq6/3
  Tiempo Disparo1/1 -> Arranq6/2
  C15/1 -> Arranq3/1
  C14/1 -> Arranq3/3
  Arranq3/1 -> Discrete-Time Integrator/1
  Condicion arranque1/1 -> Arranq3/2, Discrete-Time Integrator/2
  Pick-Up/1 -> Condicion arranque1/2
  Discrete-Time Integrator/1 -> Tiempo Disparo1/1
  Logical Operator4/1 -> Trip/1
  Entrada/1 -> Condicion arranque1/1
  T.O./1 -> Tiempo Disparo1/2

== system IEEE34BARRAS/RL5/Timer Proteccion 51 ==
  Entrada : Inport
  Pick-Up : Inport  Port=2
  T.O. : Inport  Port=3
  Arranq3 : Switch  Criteria=u2 ~= 0  Threshold=Ip1
  Arranq6 : Switch  Criteria=u2 ~= 0  Threshold=Ip1  ZeroCross=off
  C14 : Constant  Value=0
  C15 : Constant
  C16 : Constant
  Condicion arranque1 : RelationalOperator  Operator=>  OutDataTypeStr=boolean  RndMeth=Nearest
  Discrete-Time Integrator : DiscreteIntegrator  gainval=1  ExternalReset=falling  SampleTime=-1  ICPrevOutput=DiscIntNeverNeededParam  ICPrevScaledInput=DiscIntNeverNeededParam
  Logical Operator4 : Logic  Operator=NOT  AllPortsSameDT=off  OutDataTypeStr=boolean
  Tiempo Disparo1 : RelationalOperator  OutDataTypeStr=boolean  RndMeth=Nearest
  Trip : Outport
  wires:
  C16/1 -> Arranq6/1
  Arranq6/1 -> Logical Operator4/1, Arranq6/3
  Tiempo Disparo1/1 -> Arranq6/2
  T.O./1 -> Tiempo Disparo1/2
  C15/1 -> Arranq3/1
  C14/1 -> Arranq3/3
  Arranq3/1 -> Discrete-Time Integrator/1
  Condicion arranque1/1 -> Arranq3/2, Discrete-Time Integrator/2
  Pick-Up/1 -> Condicion arranque1/2
  Entrada/1 -> Condicion arranque1/1
  Discrete-Time Integrator/1 -> Tiempo Disparo1/1
  Logical Operator4/1 -> Trip/1

== system IEEE34BARRAS/RL1/RMS1/Hold derivative till next zero crossing ==
  note: Silvano Casoria
      | Power System Simulation Laboratory
      | IREQ, Hydro-Quebc
  note: Sample and Hold
  In : Inport
  S : Inport  Port=2
  Memory : Memory
  Switch : Switch  Threshold=0.5  SaturateOnIntegerOverflow=on  InputSameDT=on
  "   " : Outport  InitialOutput=0
  wires:
  S/1 -> Switch/2
  In/1 -> Switch/1
  Memory/1 -> Switch/3
  Switch/1 -> Memory/1, "   "/1

== system IEEE34BARRAS/RL1/RMS1/Hold derivative till next zero crossing1 ==
  note: Sample and Hold
  note: Silvano Casoria
      | Power System Simulation Laboratory
      | IREQ, Hydro-Quebc
  In : Inport
  S : Inport  Port=2
  Memory : Memory
  Switch : Switch  Threshold=0.5  SaturateOnIntegerOverflow=on  InputSameDT=on
  "   " : Outport  InitialOutput=0
  wires:
  Switch/1 -> "   "/1, Memory/1
  Memory/1 -> Switch/3
  In/1 -> Switch/1
  S/1 -> Switch/2

== system IEEE34BARRAS/RL1/RMS1/Hold derivative till next zero crossing2 ==
  note: Silvano Casoria
      | Power System Simulation Laboratory
      | IREQ, Hydro-Quebc
  note: Sample and Hold
  In : Inport
  S : Inport  Port=2
  Memory : Memory
  Switch : Switch  Threshold=0.5  SaturateOnIntegerOverflow=on  InputSameDT=on
  "   " : Outport  InitialOutput=0
  wires:
  S/1 -> Switch/2
  In/1 -> Switch/1
  Memory/1 -> Switch/3
  Switch/1 -> Memory/1, "   "/1

== system IEEE34BARRAS/RL2/RMS1/Hold derivative till next zero crossing ==
  note: Silvano Casoria
      | Power System Simulation Laboratory
      | IREQ, Hydro-Quebc
  note: Sample and Hold
  In : Inport
  S : Inport  Port=2
  Memory : Memory
  Switch : Switch  Threshold=0.5  SaturateOnIntegerOverflow=on  InputSameDT=on
  "   " : Outport  InitialOutput=0
  wires:
  S/1 -> Switch/2
  In/1 -> Switch/1
  Memory/1 -> Switch/3
  Switch/1 -> Memory/1, "   "/1

== system IEEE34BARRAS/RL2/RMS1/Hold derivative till next zero crossing1 ==
  note: Sample and Hold
  note: Silvano Casoria
      | Power System Simulation Laboratory
      | IREQ, Hydro-Quebc
  In : Inport
  S : Inport  Port=2
  Memory : Memory
  Switch : Switch  Threshold=0.5  SaturateOnIntegerOverflow=on  InputSameDT=on
  "   " : Outport  InitialOutput=0
  wires:
  Switch/1 -> "   "/1, Memory/1
  Memory/1 -> Switch/3
  In/1 -> Switch/1
  S/1 -> Switch/2

== system IEEE34BARRAS/RL2/RMS1/Hold derivative till next zero crossing2 ==
  note: Silvano Casoria
      | Power System Simulation Laboratory
      | IREQ, Hydro-Quebc
  note: Sample and Hold
  In : Inport
  S : Inport  Port=2
  Memory : Memory
  Switch : Switch  Threshold=0.5  SaturateOnIntegerOverflow=on  InputSameDT=on
  "   " : Outport  InitialOutput=0
  wires:
  S/1 -> Switch/2
  In/1 -> Switch/1
  Memory/1 -> Switch/3
  Switch/1 -> Memory/1, "   "/1

== system IEEE34BARRAS/RL3/RMS1/Hold derivative till next zero crossing ==
  note: Silvano Casoria
      | Power System Simulation Laboratory
      | IREQ, Hydro-Quebc
  note: Sample and Hold
  In : Inport
  S : Inport  Port=2
  Memory : Memory
  Switch : Switch  Threshold=0.5  SaturateOnIntegerOverflow=on  InputSameDT=on
  "   " : Outport  InitialOutput=0
  wires:
  S/1 -> Switch/2
  In/1 -> Switch/1
  Memory/1 -> Switch/3
  Switch/1 -> Memory/1, "   "/1

== system IEEE34BARRAS/RL3/RMS1/Hold derivative till next zero crossing1 ==
  note: Sample and Hold
  note: Silvano Casoria
      | Power System Simulation Laboratory
      | IREQ, Hydro-Quebc
  In : Inport
  S : Inport  Port=2
  Memory : Memory
  Switch : Switch  Threshold=0.5  SaturateOnIntegerOverflow=on  InputSameDT=on
  "   " : Outport  InitialOutput=0
  wires:
  Switch/1 -> "   "/1, Memory/1
  Memory/1 -> Switch/3
  In/1 -> Switch/1
  S/1 -> Switch/2

== system IEEE34BARRAS/RL3/RMS1/Hold derivative till next zero crossing2 ==
  note: Silvano Casoria
      | Power System Simulation Laboratory
      | IREQ, Hydro-Quebc
  note: Sample and Hold
  In : Inport
  S : Inport  Port=2
  Memory : Memory
  Switch : Switch  Threshold=0.5  SaturateOnIntegerOverflow=on  InputSameDT=on
  "   " : Outport  InitialOutput=0
  wires:
  S/1 -> Switch/2
  In/1 -> Switch/1
  Memory/1 -> Switch/3
  Switch/1 -> Memory/1, "   "/1

== system IEEE34BARRAS/RL4/RMS1/Hold derivative till next zero crossing ==
  note: Silvano Casoria
      | Power System Simulation Laboratory
      | IREQ, Hydro-Quebc
  note: Sample and Hold
  In : Inport
  S : Inport  Port=2
  Memory : Memory
  Switch : Switch  Threshold=0.5  SaturateOnIntegerOverflow=on  InputSameDT=on
  "   " : Outport  InitialOutput=0
  wires:
  S/1 -> Switch/2
  In/1 -> Switch/1
  Memory/1 -> Switch/3
  Switch/1 -> Memory/1, "   "/1
